simulink model "lab5_17a"  (R2017a)
settings: Solver=VariableStepAuto  StartTime=0.0  StopTime=10.0  RelTol=1e-3
undefined symbols (not defined in the file): Radix
libraries: dspmtrx3 x4, dspsigops x2, dspxfrm3 x2, dspvision x1, dspsnks4 x1
settings Model: Creator=Ross_admin  LastModifiedBy=Ross
settings OptimizationCC: BlockReduction=off  ConditionallyExecuteInputs=off  DefaultParameterBehavior=Inlined
settings DebuggingCC: AlgebraicLoopMsg=error
settings HardwareCC: ProdBitPerPointer=32  ProdBitPerSizeT=32  ProdBitPerPtrDiffT=32  ProdLargestAtomicFloat=None  ProdIntDivRoundTo=Undefined  ProdEndianess=Unspecified  ProdWordSize=32  ProdHWDeviceType=ASIC/FPGA->ASIC/FPGA  TargetBitPerPointer=64  TargetBitPerSizeT=64  TargetBitPerPtrDiffT=64  TargetLongLongMode=on  TargetIntDivRoundTo=Zero  TargetEndianess=LittleEndian  TargetWordSize=64  TargetHWDeviceType=Custom Processor->MATLAB Host Computer  ProdEqTarget=off

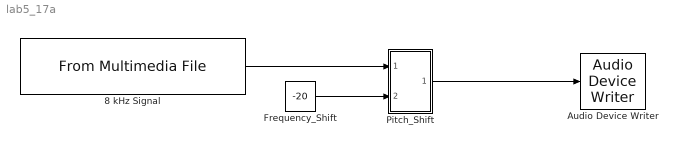
== system lab5_17a ==
  8 kHz Signal : dspvision/From Multimedia File  inputFilename=SpeechDFT-16-8-mono-5secs.wav  loop=on  numPlays=1  outputStreams=Audio only  videoDataType=single  audioDataType=double  inheritSampleTime=on  userDefinedSampleTime=1/30  noAudioOutput=off  isIntensityVideo=off  fourcc=RGB  colorVideoFormat=Separate color signals  outputEOF=off  dataOrg=Column-major  audioFrameSize=1024  computeAudioFrameSize=off  outSamplingMode=Sample based
      settings: SourceProductBaseCode=VP
  Audio Device Writer : dspsnks4/Audio Device Writer  Driver=DirectSound  Device=Default  InheritSampleRate=on  SampleRate=44100  BitDepth=16-bit integer  BufferSize=4096  NumBuffers=10  DefaultOutputChannelMapping=on  OutputChannelMapping=1:2  OutputNumUnderrunSamples=off  DriverIdx=1  DeviceWarnFlag=''
  Frequency_Shift : Constant  Value=-20  OutDataTypeStr=int16
  Pitch_Shift : Subsystem
  wires:
  8 kHz Signal/1 -> Pitch_Shift/1(In1)
  Frequency_Shift/1 -> Pitch_Shift/2(In2)
  Pitch_Shift/1(Out1) -> Audio Device Writer/1

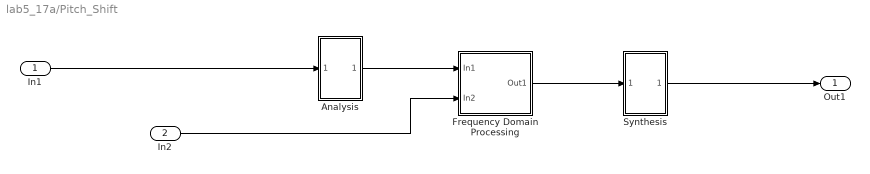
== system lab5_17a/Pitch_Shift ==
  In1 : Inport
  In2 : Inport  Port=2
  Analysis : Subsystem
  Frequency Domain Processing : Subsystem
  Synthesis : Subsystem
  Out1 : Outport
  wires:
  In1/1 -> Analysis/1(In1)
  Synthesis/1(Out1) -> Out1/1
  Frequency Domain Processing/1(Out1) -> Synthesis/1(In1)
  In2/1 -> Frequency Domain Processing/2(In2)
  Analysis/1(Out1) -> Frequency Domain Processing/1(In1)

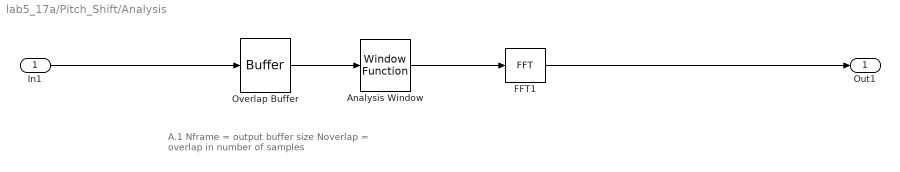
== system lab5_17a/Pitch_Shift/Analysis ==
  note: A.1
      | Nframe = output buffer size
      | Noverlap = overlap in number of samples
  In1 : Inport
  Analysis Window : dspsigops/Window Function  winmode=Apply window to input  wintype=Hanning  sampmode=Continuous  samptime=1  N=64  Rs=50  beta=10  winsamp=Periodic  UserWindow=hamming  OptParams=off  UserParams={1.0}  dataType=double  isSigned=on  wordLen=16  udDataType=sfix(16)  fracBitsMode=Best precision  numFracBits=15  roundingMode=Floor  overflowMode=off  numSidelobes=4  sidelobeLevel=-30
      settings: SourceProductName=DSP System Toolbox  SourceProductBaseCode=DS
  FFT1 : dspxfrm3/FFT  FFTImplementation=Radix-2  CompMethod=Table lookup  TableOpt=NEW  TableOptActive=Speed  BitRevOrder=off  Normalize=off  InheritFFTLength=on  FFTLength=64  WrapInput=on  roundingMode=Floor  overflowMode=off  firstCoeffMode=Specify word length  firstCoeffWordLength=16  firstCoeffFracLength=15  firstCoeffDataTypeStr=fixdt(1,16)  firstCoeffLastDataTypeStr=fixdt(1,16)  accumDataTypeStr=Inherit: Same as product output  accumLastDataTypeStr=Inherit: Same as product output  outputMin=[]  outputMax=[]
  Overlap Buffer : Buffer  N=1024  V=1024 * 3/4  OutputFrames=off
  Out1 : Outport
  wires:
  In1/1 -> Overlap Buffer/1
  Overlap Buffer/1 -> Analysis Window/1
  Analysis Window/1 -> FFT1/1
  FFT1/1 -> Out1/1

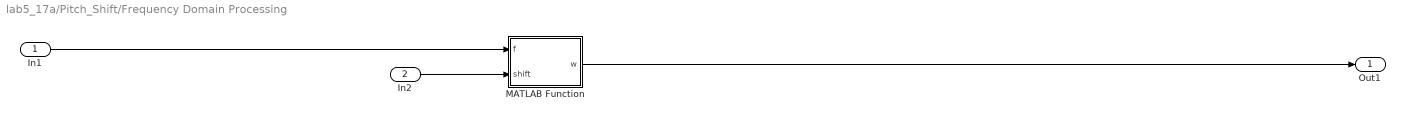
== system lab5_17a/Pitch_Shift/Frequency Domain Processing ==
  In1 : Inport
  In2 : Inport  Port=2
  MATLAB Function : MATLAB Function  TreatAsAtomicUnit=on
  Out1 : Outport
  wires:
  In1/1 -> MATLAB Function/1(f)
  In2/1 -> MATLAB Function/2(shift)
  MATLAB Function/1(w) -> Out1/1

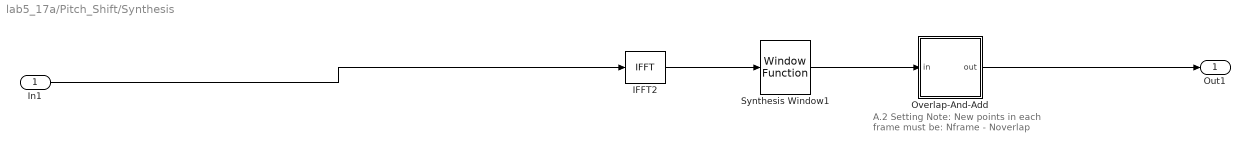
== system lab5_17a/Pitch_Shift/Synthesis ==
  note: A.2
      | Setting Note:
      | New points in each frame must be:
      | Nframe - Noverlap
  In1 : Inport
  IFFT2 : dspxfrm3/IFFT  FFTImplementation=Radix-2  CompMethod=Table lookup  TableOpt=HYBRID  TableOptActive=Speed  BitRevOrder=off  cs_in=on  Normalize=on  InheritFFTLength=on  FFTLength=64  WrapInput=on  mode=Complex  outSamplingMode=Sample based  roundingMode=Floor  overflowMode=off  firstCoeffMode=User-defined  firstCoeffWordLength=16  firstCoeffFracLength=15  firstCoeffDataTypeStr=fixdt(1,16)  firstCoeffLastDataTypeStr=fixdt(1,16)  accumDataTypeStr=Inherit: Same as product output  accumLastDataTypeStr=Inherit: Same as product output  outputMin=[]  outputMax=[]
      settings: SourceProductName=DSP System Toolbox
  Overlap-And-Add : Subsystem  mask(Overlap-And-Add){L=1024 * 1/4}
      mask prompts: L "Number of new points in each frame"
      mask help: Performs overlap-and-add on the input signal. Disjoint frames of the input signal are overlapped with each other for a specified number of points and summed.
      mask Display: disp('Overlap\nAnd\nAdd')
  Synthesis Window1 : dspsigops/Window Function  winmode=Apply window to input  wintype=Hanning  sampmode=Continuous  samptime=1  N=64  Rs=50  beta=10  winsamp=Periodic  UserWindow=hamming  OptParams=off  UserParams={1.0}  dataType=double  isSigned=on  wordLen=16  udDataType=sfix(16)  fracBitsMode=Best precision  numFracBits=15  roundingMode=Floor  overflowMode=off  numSidelobes=4  sidelobeLevel=-30
      settings: SourceProductName=DSP System Toolbox  SourceProductBaseCode=DS
  Out1 : Outport
  wires:
  IFFT2/1 -> Synthesis Window1/1
  Synthesis Window1/1 -> Overlap-And-Add/1(in)
  Overlap-And-Add/1(out) -> Out1/1
  In1/1 -> IFFT2/1

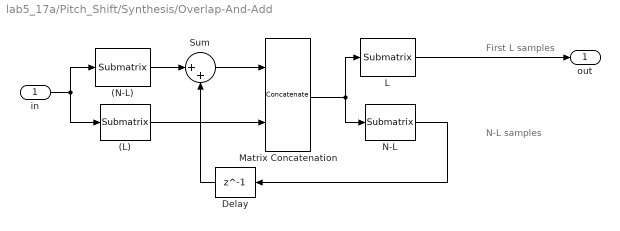
== system lab5_17a/Pitch_Shift/Synthesis/Overlap-And-Add ==
  note: First L samples
  note: N-L samples
  in : Inport
  (L) : dspmtrx3/Submatrix  RowSpan=Range of rows  RowStartMode=Offset from last  RowStartIndex=L-1  RowEndMode=Last  RowEndIndex=1  ColSpan=All columns  ColStartMode=First  ColStartIndex=1  ColEndMode=Last  ColEndIndex=1
  (N-L) : dspmtrx3/Submatrix  RowSpan=Range of rows  RowStartMode=First  RowStartIndex=1  RowEndMode=Offset from last  RowEndIndex=L  ColSpan=All columns  ColStartMode=First  ColStartIndex=1  ColEndMode=Last  ColEndIndex=1
  Delay : Delay  DelayLength=1  InitialCondition=0
  L : dspmtrx3/Submatrix  RowSpan=Range of rows  RowStartMode=First  RowStartIndex=1  RowEndMode=Index  RowEndIndex=L  ColSpan=All columns  ColStartMode=First  ColStartIndex=1  ColEndMode=Last  ColEndIndex=1
  Matrix Concatenation : Concatenate  Mode=Multidimensional array
  N-L : dspmtrx3/Submatrix  RowSpan=Range of rows  RowStartMode=Index  RowStartIndex=L+1  RowEndMode=Last  RowEndIndex=1  ColSpan=All columns  ColStartMode=First  ColStartIndex=1  ColEndMode=Last  ColEndIndex=1
  Sum : Sum  Inputs=|++  SaturateOnIntegerOverflow=on  InputSameDT=on  OutDataTypeStr=Inherit: Same as first input
  out : Outport
  wires:
  L/1 -> out/1
  Sum/1 -> Matrix Concatenation/1
  (N-L)/1 -> Sum/1
  Delay/1 -> Sum/2
  (L)/1 -> Matrix Concatenation/2
  Matrix Concatenation/1 -> L/1, N-L/1
  in/1 -> (L)/1, (N-L)/1
  N-L/1 -> Delay/1

== matlab function lab5_17a/Pitch_Shift/Frequency Domain Processing/MATLAB Function ==
  data: f input; w output; shift input
function w = fcn(f,shift)

N = length(f);
w = complex(zeros(N,1));

if shift == 0
    w = f;
else
    
    zf = f(1);            % dc term
    pf = f(2:N/2);        % positive frequencies
    lf = f(N/2 + 1);      % last positive frequency
    nf = f(N/2 + 2:N);  % negative frequencies (paired with positive frequencies)
    
    w(1) = zf;
    w(N/2+1) = complex(0);                   % just zero frequency at -pi since both positive and negative frequencies map here when shifted
        
    if shift > 0  % increase the frequencies
        
        for i=1:shift
            w(i) = complex(0);                   % fill in vacated positive frequencies with zeros
        end
        w(shift+1:N/2) = pf(1:end-shift+1);      % shift positive frequencies to the right

        w(N/2+2:end-shift) = nf(shift + 1:end);  % shift negative frequencies to the left
        for i=N-shift+1:N
            w(i) = complex(0);                   % fill in vacated negative frequencies with zeros
        end
        
    end
    if shift < 0  % decrease the frequencies
      
        nshift = abs(shift);
        
        w(2:N/2-nshift) = pf(nshift+1:end);      % shift positive frequencies to the left
        for i=N/2-nshift+2:N/2+1
            w(i) = complex(0);                   % fill in vacated positive frequencies with zeros
        end
        
        w(N/2+2+nshift:N) = nf(1:end-nshift);      % shift negative frequencies to the right
        for i=N/2+2:N/2+2+nshift-1
            w(i) = complex(0);                   % fill in vacated negative frequencies with zeros
        end
        


    end
end
